simulink model "ch7_1st_P2"  (R2017a)
settings: Solver=ode3  StartTime=0.0  StopTime=0.5  FixedStep=.001  MaxStep=.002  RelTol=1e-3  EnableMultiTasking=on
settings Model: Creator=wintersj  LastModifiedBy=wintersj
settings DataIOCC: LimitDataPoints=on  SaveFormat=Array  SignalLoggingSaveFormat=ModelDataLogs
settings OptimizationCC: ExpressionDepthLimit=2147483647  LifeSpan=inf
settings DebuggingCC: UnderspecifiedInitializationDetection=Classic  MergeDetectMultiDrivingBlocksExec=none  MaxConsecutiveZCsMsg=none  SolverPrmCheckMsg=warning  FcnCallInpInsideContextMsg=warning  StateNameClashWarn=warning  SFUnexpectedBacktrackingDiag=warning  SFNoUnconditionalDefaultTransitionDiag=warning  SFExecutionAtInitializationDiag=none
settings HardwareCC: ProdBitPerPointer=32  ProdBitPerSizeT=32  ProdBitPerPtrDiffT=32  ProdLargestAtomicFloat=None  ProdIntDivRoundTo=Undefined  ProdEndianess=Unspecified  ProdWordSize=32  ProdHWDeviceType=32-bit Generic
settings ModelReferenceCC: PropagateSignalLabelsOutOfModel=off
settings GRTTargetCC: TargetLangStandard=C89/C90 (ANSI)  GeneratePreprocessorConditionals=Disable all  CombineOutputUpdateFcns=off  GRTInterface=on
settings ConfigComp: CovMetricSettings=dw  CovHtmlReporting=on  CovSaveCumulativeToWorkspaceVar=on  CovSaveSingleToWorkspaceVar=on  CovExternalEMLEnable=off

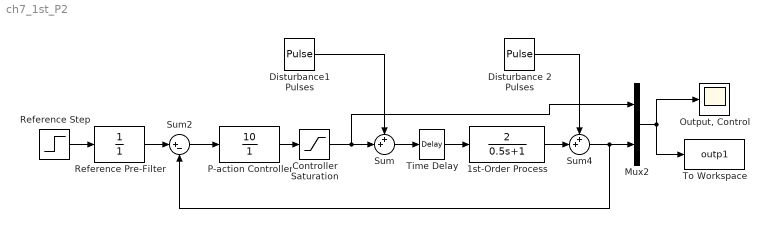
== system ch7_1st_P2 ==
  "1st-Order Process " : TransferFcn  Numerator=[2]  Denominator=[0 0.5 1]
  Controller Saturation : Saturate  UpperLimit=10  LowerLimit=-10
  Disturbance 2 Pulses : DiscretePulseGenerator  PulseType=Time based  Amplitude=0  Period=0.3  PulseWidth=50  PhaseDelay=0.1
  Disturbance1 Pulses : DiscretePulseGenerator  PulseType=Time based  Amplitude=0  Period=0.2  PulseWidth=50  PhaseDelay=0.3
  Mux2 : Mux  Inputs=2
  "Output, Control" : Scope
  P-action Controller : TransferFcn  Numerator=[10]  Denominator=[1]
  Reference Step : Step  Time=0.6  Before=1  After=5  SampleTime=0
  Reference Pre-Filter : TransferFcn  Denominator=[1]
  Sum : Sum  Inputs=++|
  Sum2 : Sum  Inputs=|+-
  Sum4 : Sum  Inputs=++|
  Time Delay : TransportDelay  DelayTime=0.01
  To Workspace : ToWorkspace  VariableName=outp1  SampleTime=-1
  wires:
  Sum2/1 -> P-action Controller/1
  Controller Saturation/1 -> Mux2/1, Sum/2
  "1st-Order Process "/1 -> Sum4/2
  Sum4/1 -> Sum2/2, Mux2/2
  Mux2/1 -> To Workspace/1, "Output, Control"/1
  Disturbance1 Pulses/1 -> Sum/1
  Disturbance 2 Pulses/1 -> Sum4/1
  P-action Controller/1 -> Controller Saturation/1
  Sum/1 -> Time Delay/1
  Time Delay/1 -> "1st-Order Process "/1
  Reference Pre-Filter/1 -> Sum2/1
  Reference Step/1 -> Reference Pre-Filter/1
